simulink library "GAS_MASTER"  (Simulink 8.6)
settings: Solver=ode45  StartTime=0.0  StopTime=10.0  RelTol=1e-3
libraries: cdsEpicsOut x12, cdsFiltCtrl x5, cdsFilt x5, cdsTP x4, VIS_LIB x4, cdsEpicsIn x3, cdsEpicsBinIn x3, cdsFunctionCall x2
(part 2 of 2)

== system GAS_MASTER/GAS_W/O_DCCTRL/LVDTINF ==
  In1 : Inport
  GAS : cdsFilt/Subsystem  Tag=cdsFilt  Description=|
      | Purpose:                                                                                                                                                                                                                                  
      | Standard CDS IIR filter module.                                                                                                                                                                                                           
      |                                                                                                                                                                                                                                           
      | Operation:                                                                                                                                                                                                                                
      | Consists of 10 second order section IIR filters, plus a ramped gain stage. In FE code, also provides pre-defined test points and excitation channel inputs. The filter coefficients are defined in the LIGO system using the 'foton' tool.
      |                                                                                                                                                                                                                                           
      | Usage:                                                                                                                                                                                                                                    
      | Name the part with the desired filter module name.
      settings: AttributesFormatString=%<Tag>
  Out1 : Outport
  wires:
  GAS/1 -> Out1/1
  In1/1 -> GAS/1

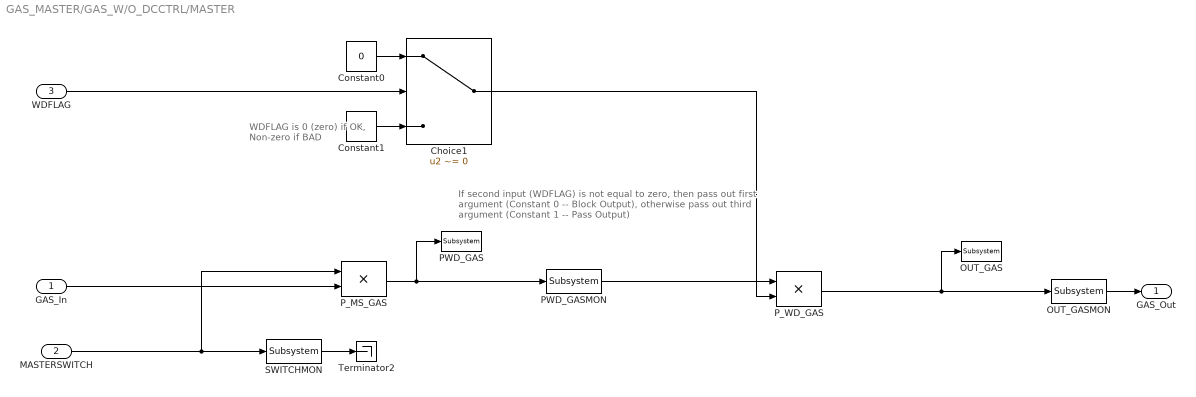
== system GAS_MASTER/GAS_W/O_DCCTRL/MASTER ==
  note: If second input (WDFLAG) is not equal to zero,
      | then pass out first argument (Constant 0 -- Block Output),
      | otherwise pass out third argument (Constant 1 -- Pass Output)
  note: WDFLAG is 0 (zero) if OK,
      | Non-zero if BAD
  GAS_In : Inport
  MASTERSWITCH : Inport  Port=2
  WDFLAG : Inport  Port=3
  Choice1 : Switch  Criteria=u2 ~= 0  Threshold=0.5
  Constant0 : Constant  Value=0
  Constant1 : Constant
  OUT_GAS : cdsTP/Subsystem  Tag=Test Point
      settings: AttributesFormatString=%<Tag>
  OUT_GASMON : cdsEpicsOut/Subsystem  Tag=cdsEpicsOutput  Description=|
      | Purpose:                                          
      | Output a FE signal to an EPICS channel.           
      |                                                   
      | Operation:                                        
      | Takes input value and passes it to EPICS record.  
      |                                                   
      | Usage:                                            
      | Name the part with the desired EPICS rrecord name.
      settings: AttributesFormatString=%<Tag>
  PWD_GAS : cdsTP/Subsystem  Tag=Test Point
      settings: AttributesFormatString=%<Tag>
  PWD_GASMON : cdsEpicsOut/Subsystem  Tag=cdsEpicsOutput  Description=|
      | Purpose:                                          
      | Output a FE signal to an EPICS channel.           
      |                                                   
      | Operation:                                        
      | Takes input value and passes it to EPICS record.  
      |                                                   
      | Usage:                                            
      | Name the part with the desired EPICS rrecord name.
      settings: AttributesFormatString=%<Tag>
  P_MS_GAS : Product  RndMeth=Zero
  P_WD_GAS : Product  RndMeth=Zero
  SWITCHMON : cdsEpicsOut/Subsystem  Tag=cdsEpicsOutput  Description=|
      | Purpose:                                          
      | Output a FE signal to an EPICS channel.           
      |                                                   
      | Operation:                                        
      | Takes input value and passes it to EPICS record.  
      |                                                   
      | Usage:                                            
      | Name the part with the desired EPICS rrecord name.
      settings: AttributesFormatString=%<Tag>
  Terminator2 : Terminator
  GAS_Out : Outport
  wires:
  SWITCHMON/1 -> Terminator2/1
  GAS_In/1 -> P_MS_GAS/2
  MASTERSWITCH/1 -> SWITCHMON/1, P_MS_GAS/1
  OUT_GASMON/1 -> GAS_Out/1
  P_MS_GAS/1 -> PWD_GAS/1, PWD_GASMON/1
  P_WD_GAS/1 -> OUT_GASMON/1, OUT_GAS/1
  Constant1/1 -> Choice1/3
  Constant0/1 -> Choice1/1
  WDFLAG/1 -> Choice1/2
  PWD_GASMON/1 -> P_WD_GAS/1
  Choice1/1 -> P_WD_GAS/2

== system GAS_MASTER/GAS_W/O_DCCTRL/TEST ==
  GAS : cdsFilt/Subsystem  Tag=cdsFilt  Description=|
      | Purpose:                                                                                                                                                                                                                                  
      | Standard CDS IIR filter module.                                                                                                                                                                                                           
      |                                                                                                                                                                                                                                           
      | Operation:                                                                                                                                                                                                                                
      | Consists of 10 second order section IIR filters, plus a ramped gain stage. In FE code, also provides pre-defined test points and excitation channel inputs. The filter coefficients are defined in the LIGO system using the 'foton' tool.
      |                                                                                                                                                                                                                                           
      | Usage:                                                                                                                                                                                                                                    
      | Name the part with the desired filter module name.
      settings: AttributesFormatString=%<Tag>
  Ground1 : Ground
  Ground7 : Ground
  STATUS : cdsEpicsBinIn/Subsystem  Tag=cdsEpicsBinIn  Description=|
      | Purpose:                                                                            
      | Create an EPICS binary (0 or 1) input channel to the FE realtime controls.          
      |                                                                                     
      | Operation:                                                                          
      | Outputs value from an EPICS ai record. Value is binary input (bi Epics record type).
      |                                                                                     
      | Usage:                                                                              
      | Name the part with the desired EPICS channel name.
      settings: AttributesFormatString=%<Tag>
  F0_Out : Outport
  wires:
  GAS/1 -> F0_Out/1
  Ground1/1 -> GAS/1
  Ground7/1 -> STATUS/1
